simulink model "projeto_final_sem_ruido"  (R2019a)
settings: Solver=FixedStepAuto  StartTime=0.0  StopTime=3  FixedStep=1e-6  RelTol=1e-3
libraries: dsparch4 x6, commsynccomp2 x1
settings Model: Creator=marco  LastModifiedBy=marco

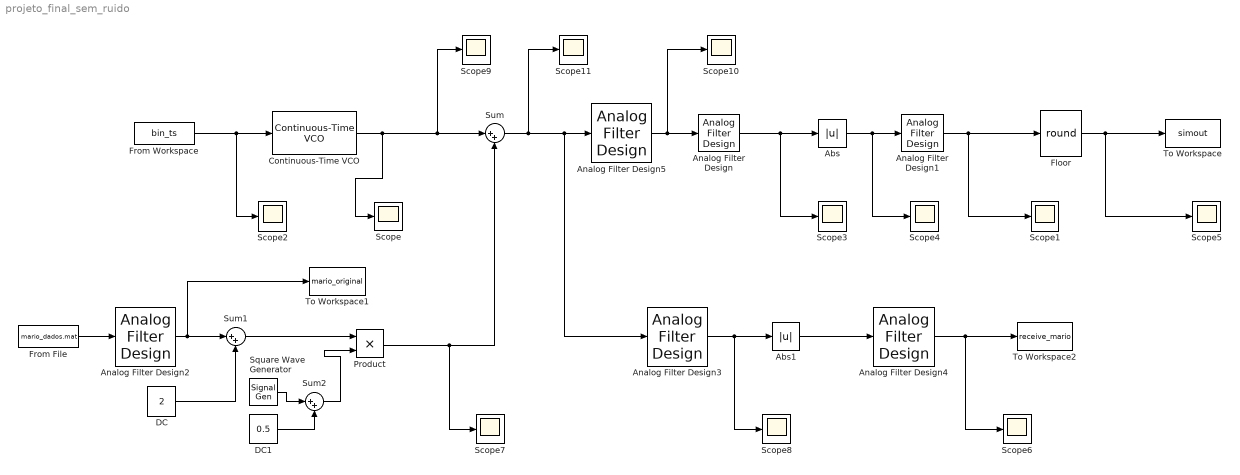
== system projeto_final_sem_ruido ==
  Abs : Abs
  Abs1 : Abs
  Analog Filter Design : dsparch4/Analog Filter Design  method=Butterworth  filttype=Bandpass  N=8  Wlo=2*pi*(1e4-2.3e3+2.9e3)  Whi=2*pi*(1e4+2.3e3+2.9e3)  Rp=2  Rs=40
  Analog Filter Design1 : dsparch4/Analog Filter Design  method=Butterworth  filttype=Lowpass  N=8  Wlo=2*pi*2e3  Whi=80  Rp=2  Rs=40
  Analog Filter Design2 : dsparch4/Analog Filter Design  method=Butterworth  filttype=Lowpass  N=10  Wlo=2*pi*5e3  Whi=2*pi*1020e3  Rp=2  Rs=40
  Analog Filter Design3 : dsparch4/Analog Filter Design  method=Butterworth  filttype=Highpass  N=10  Wlo=2*pi*5e4  Whi=2*pi*108e3  Rp=2  Rs=40
  Analog Filter Design4 : dsparch4/Analog Filter Design  method=Butterworth  filttype=Lowpass  N=10  Wlo=2*pi*30e3  Whi=2*pi*1020e3  Rp=2  Rs=40
  Analog Filter Design5 : dsparch4/Analog Filter Design  method=Butterworth  filttype=Lowpass  N=10  Wlo=2*pi*0.15e5  Whi=2*pi*108e3  Rp=2  Rs=40
  Continuous-Time VCO : commsynccomp2/Continuous-Time VCO  Ac=1  Fc=1e4  Kc=0.1e4  Ph=0
      settings: SourceProductName=Communications Toolbox  SourceProductBaseCode=CM
  DC : Constant  Value=2
  DC1 : Constant  Value=0.5
  Floor : Rounding  Operator=round
  From Workspace : FromWorkspace  VariableName=bin_ts  OutDataTypeStr=double  SampleTime=0  Interpolate=off  OutputAfterFinalValue=Setting to zero
  From File : FromFile  FileName=mario_dados.mat  SampleTime=0  ExtrapolationBeforeFirstDataPoint=Ground value
  Product : Product
  Scope{,1..11} (12 alike) : Scope
  Square Wave Generator : SignalGenerator  WaveForm=square  Amplitude=0.5  Frequency=105e3
  Sum : Sum  Inputs=|++
  Sum1 : Sum  Inputs=|++
  Sum2 : Sum  Inputs=|++
  To Workspace : ToWorkspace  VariableName=simout  SaveFormat=Timeseries  SampleTime=-1
  To Workspace1 : ToWorkspace  VariableName=mario_original  SaveFormat=Timeseries  SampleTime=1e-5
  To Workspace2 : ToWorkspace  VariableName=receive_mario  SaveFormat=Timeseries  SampleTime=1e-5
  wires:
  Continuous-Time VCO/1 -> Scope9/1, Sum/1, Scope/1
  Abs/1 -> Scope4/1, Analog Filter Design1/1
  Analog Filter Design/1 -> Scope3/1, Abs/1
  From Workspace/1 -> Scope2/1, Continuous-Time VCO/1
  Floor/1 -> Scope5/1, To Workspace/1
  Analog Filter Design2/1 -> To Workspace1/1, Sum1/1
  Square Wave Generator/1 -> Sum2/1
  From File/1 -> Analog Filter Design2/1
  Sum2/1 -> Product/2
  DC/1 -> Sum1/2
  Sum1/1 -> Product/1
  DC1/1 -> Sum2/2
  Sum/1 -> Scope11/1, Analog Filter Design5/1, Analog Filter Design3/1
  Analog Filter Design3/1 -> Scope8/1, Abs1/1
  Analog Filter Design4/1 -> Scope6/1, To Workspace2/1
  Abs1/1 -> Analog Filter Design4/1
  Product/1 -> Scope7/1, Sum/2
  Analog Filter Design5/1 -> Scope10/1, Analog Filter Design/1
  Analog Filter Design1/1 -> Floor/1, Scope1/1
